simulink model "fuzzy"  (R2020b)
settings: Solver=VariableStepAuto  StartTime=0.0  StopTime=5000  RelTol=1e-3
values from neighbouring files (symbols this model uses):
  A = [-0.0019 0.0024 -0.0009;-0.0034 -0.0043 -0.0008;-0.0009 -0.0052 -0.0055]    [Paperwork.m]    (also in chapter6.m; chapter8.m = [a11 0.0024 -0.0009;-0.0034 a22 a23;-0.0009 -0.0052 a33]; fuzzy_data.m)
  B = [0.0003 0.0013 -0.0566; -0.0005 0.0019 -0.0822; 0.0025 0.0067 -0.2818]    [Paperwork.m]    (also in chapter6.m; chapter8.m; fuzzy_data.m)
  C = [-12.8258 4.0787 0.1685;-3.7520 -0.8266 -1.9955;-6.2674 -17.6857 -0.7129]    [Paperwork.m]    (also in chapter6.m; chapter8.m; fuzzy_data.m)
  D = zeros(3,3)    [Paperwork.m]    (also in chapter6.m; chapter8.m; fuzzy_data.m)
libraries: fuzblock x1
settings Model: Creator=Javad  LastModifiedBy=Javad

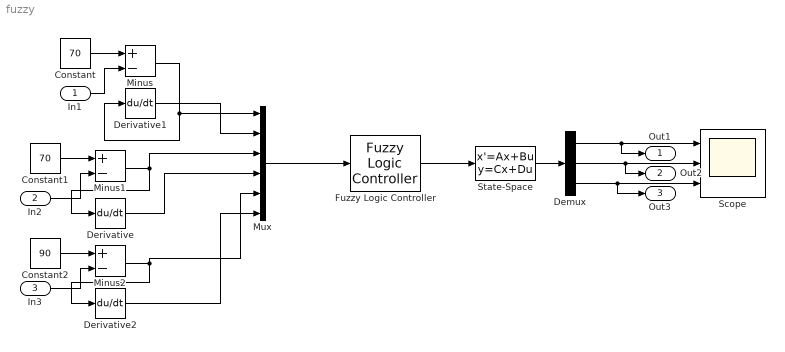
== system fuzzy ==
  In1 : Inport
  In2 : Inport  Port=2
  In3 : Inport  Port=3
  Constant : Constant  Value=70
  Constant1 : Constant  Value=70
  Constant2 : Constant  Value=90
  Demux : Demux  Outputs=3
  Derivative : Derivative
  Derivative1 : Derivative
  Derivative2 : Derivative
  Fuzzy Logic Controller : fuzblock/Fuzzy Logic  Controller  FIS='StateSpace_fuzzy.fis'  OutputSampleNumber=101  DataType=double  FuzzifiedInputs=off  RuleFiringStrengths=off  RuleOutputs=off  AggregatedOutputs=off  SimulateUsing=Interpreted execution  OutOfRangeInputValueMessage=warning  NoRuleFiredMessage=warning  EmptyOutputFuzzySetMessage=warning
  Minus : Sum  Inputs=+-
  Minus1 : Sum  Inputs=+-
  Minus2 : Sum  Inputs=+-
  Mux : Mux  Inputs=6
  Scope : Scope  NumInputPorts=3
  State-Space : StateSpace  A=A  B=B  C=C  D=D  InitialCondition=0
  Out1 : Outport
  Out2 : Outport  Port=2
  Out3 : Outport  Port=3
  wires:
  Fuzzy Logic Controller/1 -> State-Space/1
  State-Space/1 -> Demux/1
  Demux/1 -> Out1/1, Scope/1
  Demux/2 -> Out2/1, Scope/2
  Demux/3 -> Out3/1, Scope/3
  Mux/1 -> Fuzzy Logic Controller/1
  Constant/1 -> Minus/1
  Constant2/1 -> Minus2/1
  Constant1/1 -> Minus1/1
  Minus1/1 -> Mux/3, Derivative/1
  Minus/1 -> Mux/1, Derivative1/1
  Minus2/1 -> Mux/5, Derivative2/1
  Derivative2/1 -> Mux/6
  Derivative/1 -> Mux/4
  Derivative1/1 -> Mux/2
  In1/1 -> Minus/2
  In2/1 -> Minus1/2
  In3/1 -> Minus2/2
